simulink model "AM_DSB_LC"  (R2024a)
settings: Solver=VariableStepAuto  StartTime=0.0  StopTime=10.0  RelTol=1e-3
settings Model: Creator=zeyad  LastModifiedBy=zeyad

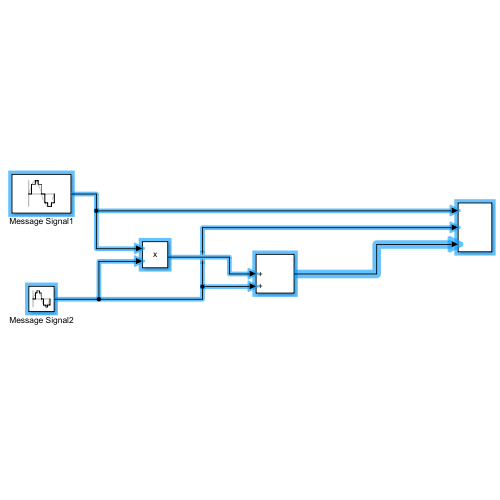
[thumbnail: Simulink's stored preview of the top-level diagram]
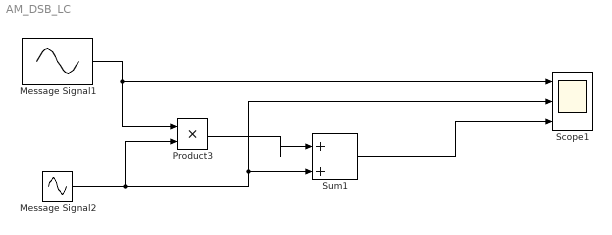
== system AM_DSB_LC ==
  Message Signal1 : Sin  Frequency=5  SampleTime=1/1000
  Message Signal2 : Sin  Frequency=50  SampleTime=1/1000
  Product3 : Product
  Scope1 : Scope  NumInputPorts=3
  Sum1 : Sum  Inputs=|++
  wires:
  Message Signal2/1 -> Product3/2, Scope1/2, Sum1/2
  Message Signal1/1 -> Product3/1, Scope1/1
  Product3/1 -> Sum1/1
  Sum1/1 -> Scope1/3
